simulink library "GAS_MODAL_MASTER"  (Simulink 8.6)
settings: Solver=VariableStepAuto  StartTime=0.0  StopTime=10.0  RelTol=1e-3
libraries: cdsEpicsOut x7, cdsFilt x5, cdsFiltCtrl x3, cdsEpicsIn x2, cdsTP x2, cdsEpicsBinIn x2, VIS_LIB x2, cdsFunctionCall x1
settings Model: Creator=controls  LastModifiedBy=controls

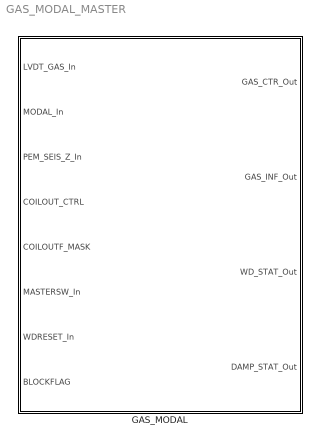
== system GAS_MODAL_MASTER ==
  GAS_MODAL : Subsystem

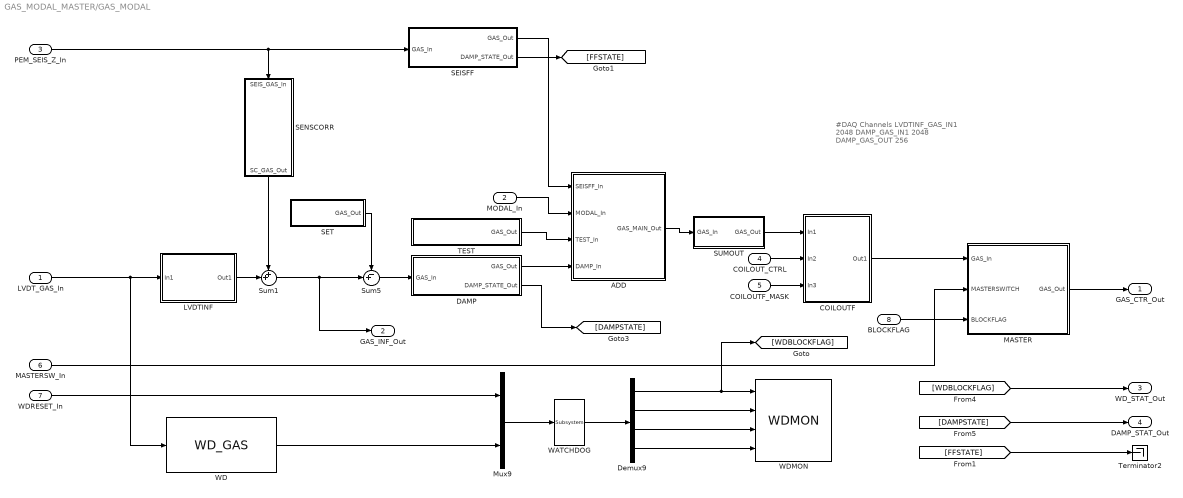
== system GAS_MODAL_MASTER/GAS_MODAL ==
  note: #DAQ Channels
      | LVDTINF_GAS_IN1 2048
      | DAMP_GAS_IN1 2048
      | DAMP_GAS_OUT 256
  LVDT_GAS_In : Inport
  MODAL_In : Inport  Port=2
  PEM_SEIS_Z_In : Inport  Port=3
  COILOUT_CTRL : Inport  Port=4
  COILOUTF_MASK : Inport  Port=5
  MASTERSW_In : Inport  Port=6
  WDRESET_In : Inport  Port=7
  BLOCKFLAG : Inport  Port=8
  ADD : Subsystem
  COILOUTF : Subsystem
  DAMP : Subsystem
  Demux9 : Demux
  LVDTINF : Subsystem
  MASTER : Subsystem
  Mux9 : Mux  Inputs=2
  SEISFF : Subsystem
  SENSCORR : Subsystem
  SET : Subsystem
  SUMOUT : Subsystem
  Sum1 : Sum  Inputs=++|
  Sum5 : Sum  Inputs=-+|
  TEST : Subsystem
  Terminator2 : Terminator
  WATCHDOG : cdsFunctionCall/Subsystem  Tag=cdsFunctionCall  Description=inline OSEMWATCHDOG /opt/rtcds/userapps/release/vis/common/src/WATCHDOG.c
      settings: AttributesFormatString=%<Tag>\n%<Description>
  WD : VIS_LIB/WD_GAS
  WDMON : VIS_LIB/WDMON
  GAS_CTR_Out : Outport
  GAS_INF_Out : Outport  Port=2
  WD_STAT_Out : Outport  Port=3
  DAMP_STAT_Out : Outport  Port=4
  wires:
  WDRESET_In/1 -> Mux9/1
  COILOUTF_MASK/1 -> COILOUTF/3(In3)
  COILOUT_CTRL/1 -> COILOUTF/2(In2)
  LVDT_GAS_In/1 -> WD/1, LVDTINF/1(In1)
  Demux9/1 -> WDMON/1, [WDBLOCKFLAG]
  ADD/1(GAS_MAIN_Out) -> SUMOUT/1(GAS_In)
  MASTER/1(GAS_Out) -> GAS_CTR_Out/1
  BLOCKFLAG/1 -> MASTER/3(BLOCKFLAG)
  TEST/1(GAS_Out) -> ADD/3(TEST_In)
  [DAMPSTATE] -> DAMP_STAT_Out/1
  [WDBLOCKFLAG] -> WD_STAT_Out/1
  MASTERSW_In/1 -> MASTER/2(MASTERSWITCH)
  DAMP/1(GAS_Out) -> ADD/4(DAMP_In)
  DAMP/2(DAMP_STATE_Out) -> [DAMPSTATE]
  Mux9/1 -> WATCHDOG/1
  Demux9/4 -> WDMON/4
  WATCHDOG/1 -> Demux9/1
  LVDTINF/1(Out1) -> Sum1/2
  COILOUTF/1(Out1) -> MASTER/1(GAS_In)
  WD/1 -> Mux9/2
  Demux9/3 -> WDMON/3
  Demux9/2 -> WDMON/2
  MODAL_In/1 -> ADD/2(MODAL_In)
  Sum5/1 -> DAMP/1(GAS_In)
  SET/1(GAS_Out) -> Sum5/1
  SUMOUT/1(GAS_Out) -> COILOUTF/1(In1)
  SENSCORR/1(SC_GAS_Out) -> Sum1/1
  Sum1/1 -> GAS_INF_Out/1, Sum5/2
  PEM_SEIS_Z_In/1 -> SENSCORR/1(SEIS_GAS_In), SEISFF/1(GAS_In)
  SEISFF/2(DAMP_STATE_Out) -> [FFSTATE]
  SEISFF/1(GAS_Out) -> ADD/1(SEISFF_In)
  [FFSTATE] -> Terminator2/1

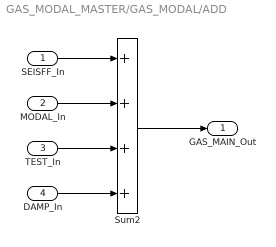
== system GAS_MODAL_MASTER/GAS_MODAL/ADD ==
  SEISFF_In : Inport
  MODAL_In : Inport  Port=2
  TEST_In : Inport  Port=3
  DAMP_In : Inport  Port=4
  Sum2 : Sum  Inputs=++++
  GAS_MAIN_Out : Outport
  wires:
  Sum2/1 -> GAS_MAIN_Out/1
  MODAL_In/1 -> Sum2/2
  TEST_In/1 -> Sum2/3
  DAMP_In/1 -> Sum2/4
  SEISFF_In/1 -> Sum2/1

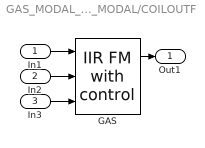
== system GAS_MODAL_MASTER/GAS_MODAL/COILOUTF ==
  In1 : Inport
  In2 : Inport  Port=2
  In3 : Inport  Port=3
  GAS : cdsFiltCtrl/IIR FM with control  Tag=cdsFiltCtrl  Description=|
      | cdsFiltCntrl is the standard IIR filter module (exactly the same as cdsFilt) but with added control data output 'Ctrl'. Filter module digital signal output appears on the first output, which is called 'Val'. 'Ctrl' output has a bit pattern encoding the state of filter's on/off switches (FM1 through FM10). The bit values are:
      |                                                                                                                                                                                                                                                                                                                                       
      | module 	hex	dec                                                                                                                                                                                                                                                                                                                       
      | -----------------------                                                                                                                                                                                                                                                                                                               
      | FM1	0x20                    32                                                                                                                                                                                                                                                                                                        
      | FM2	0x80                     128                                                                                                                                                                                                                                                                                                      
      | FM3	0x200                   512                                                                                                                                                                                                                                                                                                       
      | FM4	0x800                   2048                                                                                                                                                                                                                                                                                                      
      | FM5	0x2000                 8192                                                                                                                                                                                                                                                                                                       
      | FM6	0x8000                 32768                                                                                                                                                                                                                                                                                                      
      | FM7	0x20000                131072                                                                                                                                                                                                                                                                                                     
      | FM8	0x80000                 524288                                                                                                                                                                                                                                                                                                    
      | FM9	0x200000               2097152                                                                                                                                                                                                                                                                                                    
      | FM10	0x800000               8388608                                                                                                                                                                                                                                                                                                   
      |                                                                                                                                                                                                                                                                                                                                       
      | This bit data can be used to drive some other switches or it can be output using a binary I/O module.
      settings: AttributesFormatString=%<Tag>
  Out1 : Outport
  wires:
  In1/1 -> GAS/1
  In3/1 -> GAS/3
  In2/1 -> GAS/2
  GAS/1 -> Out1/1

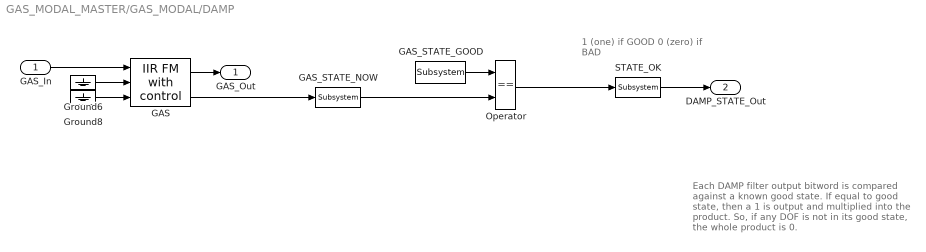
== system GAS_MODAL_MASTER/GAS_MODAL/DAMP ==
  note: Each DAMP filter output bitword is
      | compared against a known good state.
      | If equal to good state, then a 1 is output
      | and multiplied into the product. So, if any DOF
      | is not in its good state, the whole product is 0.
  note: 1 (one) if GOOD
      | 0 (zero) if BAD
  GAS_In : Inport
  GAS : cdsFiltCtrl/IIR FM with control  Tag=cdsFiltCtrl  Description=|
      | cdsFiltCntrl is the standard IIR filter module (exactly the same as cdsFilt) but with added control data output 'Ctrl'. Filter module digital signal output appears on the first output, which is called 'Val'. 'Ctrl' output has a bit pattern encoding the state of filter's on/off switches (FM1 through FM10). The bit values are:
      |                                                                                                                                                                                                                                                                                                                                       
      | module 	hex	dec                                                                                                                                                                                                                                                                                                                       
      | -----------------------                                                                                                                                                                                                                                                                                                               
      | FM1	0x20                    32                                                                                                                                                                                                                                                                                                        
      | FM2	0x80                     128                                                                                                                                                                                                                                                                                                      
      | FM3	0x200                   512                                                                                                                                                                                                                                                                                                       
      | FM4	0x800                   2048                                                                                                                                                                                                                                                                                                      
      | FM5	0x2000                 8192                                                                                                                                                                                                                                                                                                       
      | FM6	0x8000                 32768                                                                                                                                                                                                                                                                                                      
      | FM7	0x20000                131072                                                                                                                                                                                                                                                                                                     
      | FM8	0x80000                 524288                                                                                                                                                                                                                                                                                                    
      | FM9	0x200000               2097152                                                                                                                                                                                                                                                                                                    
      | FM10	0x800000               8388608                                                                                                                                                                                                                                                                                                   
      |                                                                                                                                                                                                                                                                                                                                       
      | This bit data can be used to drive some other switches or it can be output using a binary I/O module.
      settings: AttributesFormatString=%<Tag>
  GAS_STATE_GOOD : cdsEpicsIn/Subsystem  Tag=cdsEpicsIn  Description=|
      | Purpose:                                                                              
      | Create an EPICS input channel connection to the FE realtime controls.                 
      |                                                                                       
      | Operation:                                                                            
      | Outputs value from an EPICS ai record. Value is floating point with a precision of 3..
      |                                                                                       
      | Usage:                                                                                
      | Name the part with the desired EPICS channel name.
      settings: AttributesFormatString=%<Tag>
  GAS_STATE_NOW : cdsEpicsOut/Subsystem  Tag=cdsEpicsOutput  Description=|
      | Purpose:                                          
      | Output a FE signal to an EPICS channel.           
      |                                                   
      | Operation:                                        
      | Takes input value and passes it to EPICS record.  
      |                                                   
      | Usage:                                            
      | Name the part with the desired EPICS rrecord name.
      settings: AttributesFormatString=%<Tag>
  Ground6 : Ground
  Ground8 : Ground
  Operator : RelationalOperator  Operator===  OutDataTypeStr=boolean
  STATE_OK : cdsEpicsOut/Subsystem  Tag=cdsEpicsOutput  Description=|
      | Purpose:                                          
      | Output a FE signal to an EPICS channel.           
      |                                                   
      | Operation:                                        
      | Takes input value and passes it to EPICS record.  
      |                                                   
      | Usage:                                            
      | Name the part with the desired EPICS rrecord name.
      settings: AttributesFormatString=%<Tag>
  GAS_Out : Outport
  DAMP_STATE_Out : Outport  Port=2
  wires:
  Ground6/1 -> GAS/2
  GAS_In/1 -> GAS/1
  GAS/1 -> GAS_Out/1
  GAS_STATE_GOOD/1 -> Operator/1
  GAS/2 -> GAS_STATE_NOW/1
  GAS_STATE_NOW/1 -> Operator/2
  STATE_OK/1 -> DAMP_STATE_Out/1
  Ground8/1 -> GAS/3
  Operator/1 -> STATE_OK/1

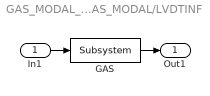
== system GAS_MODAL_MASTER/GAS_MODAL/LVDTINF ==
  In1 : Inport
  GAS : cdsFilt/Subsystem  Tag=cdsFilt  Description=|
      | Purpose:                                                                                                                                                                                                                                  
      | Standard CDS IIR filter module.                                                                                                                                                                                                           
      |                                                                                                                                                                                                                                           
      | Operation:                                                                                                                                                                                                                                
      | Consists of 10 second order section IIR filters, plus a ramped gain stage. In FE code, also provides pre-defined test points and excitation channel inputs. The filter coefficients are defined in the LIGO system using the 'foton' tool.
      |                                                                                                                                                                                                                                           
      | Usage:                                                                                                                                                                                                                                    
      | Name the part with the desired filter module name.
      settings: AttributesFormatString=%<Tag>
  Out1 : Outport
  wires:
  In1/1 -> GAS/1
  GAS/1 -> Out1/1

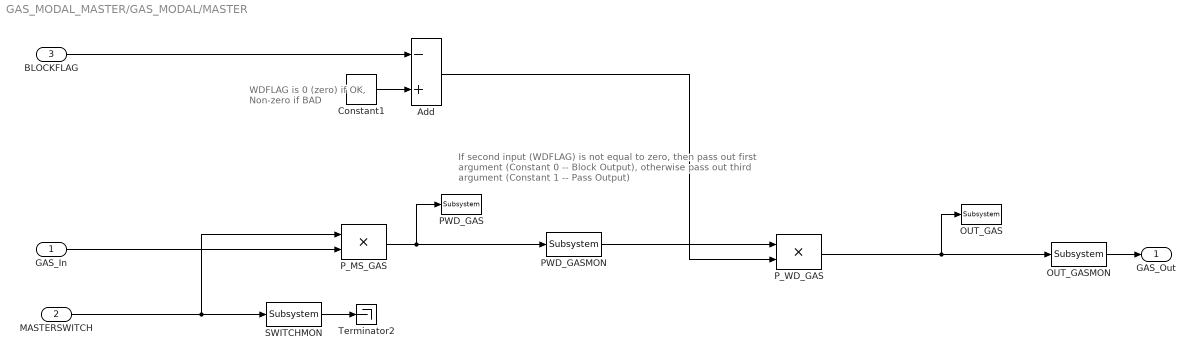
== system GAS_MODAL_MASTER/GAS_MODAL/MASTER ==
  note: WDFLAG is 0 (zero) if OK,
      | Non-zero if BAD
  note: If second input (WDFLAG) is not equal to zero,
      | then pass out first argument (Constant 0 -- Block Output),
      | otherwise pass out third argument (Constant 1 -- Pass Output)
  GAS_In : Inport
  MASTERSWITCH : Inport  Port=2
  BLOCKFLAG : Inport  Port=3
  Add : Sum  Inputs=-+
  Constant1 : Constant
  OUT_GAS : cdsTP/Subsystem  Tag=Test Point
      settings: AttributesFormatString=%<Tag>
  OUT_GASMON : cdsEpicsOut/Subsystem  Tag=cdsEpicsOutput  Description=|
      | Purpose:                                          
      | Output a FE signal to an EPICS channel.           
      |                                                   
      | Operation:                                        
      | Takes input value and passes it to EPICS record.  
      |                                                   
      | Usage:                                            
      | Name the part with the desired EPICS rrecord name.
      settings: AttributesFormatString=%<Tag>
  PWD_GAS : cdsTP/Subsystem  Tag=Test Point
      settings: AttributesFormatString=%<Tag>
  PWD_GASMON : cdsEpicsOut/Subsystem  Tag=cdsEpicsOutput  Description=|
      | Purpose:                                          
      | Output a FE signal to an EPICS channel.           
      |                                                   
      | Operation:                                        
      | Takes input value and passes it to EPICS record.  
      |                                                   
      | Usage:                                            
      | Name the part with the desired EPICS rrecord name.
      settings: AttributesFormatString=%<Tag>
  P_MS_GAS : Product  RndMeth=Zero
  P_WD_GAS : Product  RndMeth=Zero
  SWITCHMON : cdsEpicsOut/Subsystem  Tag=cdsEpicsOutput  Description=|
      | Purpose:                                          
      | Output a FE signal to an EPICS channel.           
      |                                                   
      | Operation:                                        
      | Takes input value and passes it to EPICS record.  
      |                                                   
      | Usage:                                            
      | Name the part with the desired EPICS rrecord name.
      settings: AttributesFormatString=%<Tag>
  Terminator2 : Terminator
  GAS_Out : Outport
  wires:
  Add/1 -> P_WD_GAS/2
  PWD_GASMON/1 -> P_WD_GAS/1
  BLOCKFLAG/1 -> Add/1
  Constant1/1 -> Add/2
  P_WD_GAS/1 -> OUT_GAS/1, OUT_GASMON/1
  P_MS_GAS/1 -> PWD_GASMON/1, PWD_GAS/1
  OUT_GASMON/1 -> GAS_Out/1
  MASTERSWITCH/1 -> P_MS_GAS/1, SWITCHMON/1
  GAS_In/1 -> P_MS_GAS/2
  SWITCHMON/1 -> Terminator2/1

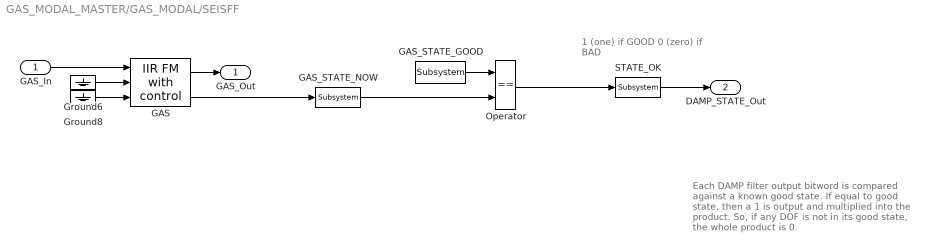
== system GAS_MODAL_MASTER/GAS_MODAL/SEISFF ==
  note: Each DAMP filter output bitword is
      | compared against a known good state.
      | If equal to good state, then a 1 is output
      | and multiplied into the product. So, if any DOF
      | is not in its good state, the whole product is 0.
  note: 1 (one) if GOOD
      | 0 (zero) if BAD
  GAS_In : Inport
  GAS : cdsFiltCtrl/IIR FM with control  Tag=cdsFiltCtrl  Description=|
      | cdsFiltCntrl is the standard IIR filter module (exactly the same as cdsFilt) but with added control data output 'Ctrl'. Filter module digital signal output appears on the first output, which is called 'Val'. 'Ctrl' output has a bit pattern encoding the state of filter's on/off switches (FM1 through FM10). The bit values are:
      |                                                                                                                                                                                                                                                                                                                                       
      | module 	hex	dec                                                                                                                                                                                                                                                                                                                       
      | -----------------------                                                                                                                                                                                                                                                                                                               
      | FM1	0x20                    32                                                                                                                                                                                                                                                                                                        
      | FM2	0x80                     128                                                                                                                                                                                                                                                                                                      
      | FM3	0x200                   512                                                                                                                                                                                                                                                                                                       
      | FM4	0x800                   2048                                                                                                                                                                                                                                                                                                      
      | FM5	0x2000                 8192                                                                                                                                                                                                                                                                                                       
      | FM6	0x8000                 32768                                                                                                                                                                                                                                                                                                      
      | FM7	0x20000                131072                                                                                                                                                                                                                                                                                                     
      | FM8	0x80000                 524288                                                                                                                                                                                                                                                                                                    
      | FM9	0x200000               2097152                                                                                                                                                                                                                                                                                                    
      | FM10	0x800000               8388608                                                                                                                                                                                                                                                                                                   
      |                                                                                                                                                                                                                                                                                                                                       
      | This bit data can be used to drive some other switches or it can be output using a binary I/O module.
      settings: AttributesFormatString=%<Tag>
  GAS_STATE_GOOD : cdsEpicsIn/Subsystem  Tag=cdsEpicsIn  Description=|
      | Purpose:                                                                              
      | Create an EPICS input channel connection to the FE realtime controls.                 
      |                                                                                       
      | Operation:                                                                            
      | Outputs value from an EPICS ai record. Value is floating point with a precision of 3..
      |                                                                                       
      | Usage:                                                                                
      | Name the part with the desired EPICS channel name.
      settings: AttributesFormatString=%<Tag>
  GAS_STATE_NOW : cdsEpicsOut/Subsystem  Tag=cdsEpicsOutput  Description=|
      | Purpose:                                          
      | Output a FE signal to an EPICS channel.           
      |                                                   
      | Operation:                                        
      | Takes input value and passes it to EPICS record.  
      |                                                   
      | Usage:                                            
      | Name the part with the desired EPICS rrecord name.
      settings: AttributesFormatString=%<Tag>
  Ground6 : Ground
  Ground8 : Ground
  Operator : RelationalOperator  Operator===  OutDataTypeStr=boolean
  STATE_OK : cdsEpicsOut/Subsystem  Tag=cdsEpicsOutput  Description=|
      | Purpose:                                          
      | Output a FE signal to an EPICS channel.           
      |                                                   
      | Operation:                                        
      | Takes input value and passes it to EPICS record.  
      |                                                   
      | Usage:                                            
      | Name the part with the desired EPICS rrecord name.
      settings: AttributesFormatString=%<Tag>
  GAS_Out : Outport
  DAMP_STATE_Out : Outport  Port=2
  wires:
  Ground6/1 -> GAS/2
  GAS_In/1 -> GAS/1
  GAS/1 -> GAS_Out/1
  GAS_STATE_GOOD/1 -> Operator/1
  GAS/2 -> GAS_STATE_NOW/1
  GAS_STATE_NOW/1 -> Operator/2
  STATE_OK/1 -> DAMP_STATE_Out/1
  Ground8/1 -> GAS/3
  Operator/1 -> STATE_OK/1

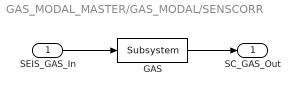
== system GAS_MODAL_MASTER/GAS_MODAL/SENSCORR ==
  SEIS_GAS_In : Inport
  GAS : cdsFilt/Subsystem  Tag=cdsFilt  Description=|
      | Purpose:                                                                                                                                                                                                                                  
      | Standard CDS IIR filter module.                                                                                                                                                                                                           
      |                                                                                                                                                                                                                                           
      | Operation:                                                                                                                                                                                                                                
      | Consists of 10 second order section IIR filters, plus a ramped gain stage. In FE code, also provides pre-defined test points and excitation channel inputs. The filter coefficients are defined in the LIGO system using the 'foton' tool.
      |                                                                                                                                                                                                                                           
      | Usage:                                                                                                                                                                                                                                    
      | Name the part with the desired filter module name.
      settings: AttributesFormatString=%<Tag>
  SC_GAS_Out : Outport
  wires:
  SEIS_GAS_In/1 -> GAS/1
  GAS/1 -> SC_GAS_Out/1

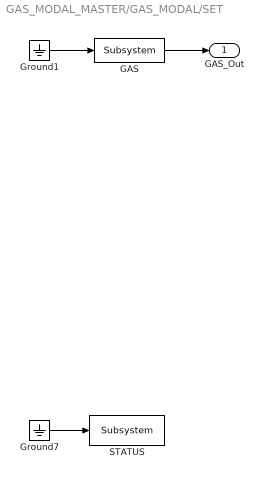
== system GAS_MODAL_MASTER/GAS_MODAL/SET ==
  GAS : cdsFilt/Subsystem  Tag=cdsFilt  Description=|
      | Purpose:                                                                                                                                                                                                                                  
      | Standard CDS IIR filter module.                                                                                                                                                                                                           
      |                                                                                                                                                                                                                                           
      | Operation:                                                                                                                                                                                                                                
      | Consists of 10 second order section IIR filters, plus a ramped gain stage. In FE code, also provides pre-defined test points and excitation channel inputs. The filter coefficients are defined in the LIGO system using the 'foton' tool.
      |                                                                                                                                                                                                                                           
      | Usage:                                                                                                                                                                                                                                    
      | Name the part with the desired filter module name.
      settings: AttributesFormatString=%<Tag>
  Ground1 : Ground
  Ground7 : Ground
  STATUS : cdsEpicsBinIn/Subsystem  Tag=cdsEpicsBinIn  Description=|
      | Purpose:                                                                            
      | Create an EPICS binary (0 or 1) input channel to the FE realtime controls.          
      |                                                                                     
      | Operation:                                                                          
      | Outputs value from an EPICS ai record. Value is binary input (bi Epics record type).
      |                                                                                     
      | Usage:                                                                              
      | Name the part with the desired EPICS channel name.
      settings: AttributesFormatString=%<Tag>
  GAS_Out : Outport
  wires:
  GAS/1 -> GAS_Out/1
  Ground1/1 -> GAS/1
  Ground7/1 -> STATUS/1

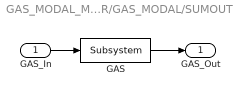
== system GAS_MODAL_MASTER/GAS_MODAL/SUMOUT ==
  GAS_In : Inport
  GAS : cdsFilt/Subsystem  Tag=cdsFilt  Description=|
      | Purpose:                                                                                                                                                                                                                                  
      | Standard CDS IIR filter module.                                                                                                                                                                                                           
      |                                                                                                                                                                                                                                           
      | Operation:                                                                                                                                                                                                                                
      | Consists of 10 second order section IIR filters, plus a ramped gain stage. In FE code, also provides pre-defined test points and excitation channel inputs. The filter coefficients are defined in the LIGO system using the 'foton' tool.
      |                                                                                                                                                                                                                                           
      | Usage:                                                                                                                                                                                                                                    
      | Name the part with the desired filter module name.
      settings: AttributesFormatString=%<Tag>
  GAS_Out : Outport
  wires:
  GAS_In/1 -> GAS/1
  GAS/1 -> GAS_Out/1

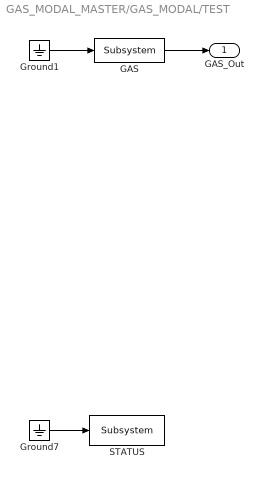
== system GAS_MODAL_MASTER/GAS_MODAL/TEST ==
  GAS : cdsFilt/Subsystem  Tag=cdsFilt  Description=|
      | Purpose:                                                                                                                                                                                                                                  
      | Standard CDS IIR filter module.                                                                                                                                                                                                           
      |                                                                                                                                                                                                                                           
      | Operation:                                                                                                                                                                                                                                
      | Consists of 10 second order section IIR filters, plus a ramped gain stage. In FE code, also provides pre-defined test points and excitation channel inputs. The filter coefficients are defined in the LIGO system using the 'foton' tool.
      |                                                                                                                                                                                                                                           
      | Usage:                                                                                                                                                                                                                                    
      | Name the part with the desired filter module name.
      settings: AttributesFormatString=%<Tag>
  Ground1 : Ground
  Ground7 : Ground
  STATUS : cdsEpicsBinIn/Subsystem  Tag=cdsEpicsBinIn  Description=|
      | Purpose:                                                                            
      | Create an EPICS binary (0 or 1) input channel to the FE realtime controls.          
      |                                                                                     
      | Operation:                                                                          
      | Outputs value from an EPICS ai record. Value is binary input (bi Epics record type).
      |                                                                                     
      | Usage:                                                                              
      | Name the part with the desired EPICS channel name.
      settings: AttributesFormatString=%<Tag>
  GAS_Out : Outport
  wires:
  Ground7/1 -> STATUS/1
  Ground1/1 -> GAS/1
  GAS/1 -> GAS_Out/1
